simulink model "ProperModel"  (R2024b)
settings: Solver=VariableStepAuto  StartTime=0.0  StopTime=10.0  RelTol=1e-3
values from neighbouring files (symbols this model uses):
  I = diag(Iv)    [InitDoubleSpin.m]    (also in InitLab03.m)
  invI = inv(I)    [InitDoubleSpin.m]    (also in InitLab03.m)
  torque = 0    [InitDoubleSpin.m]
  w0 = [1e-6; 0.005; 0.2]    [InitDoubleSpin.m]    (also in InitLab03.m = [2*pi; 0.5; 1])
  wr0 = 2*pi    (= 6.28318530718)    [InitDoubleSpin.m]
undefined symbols (not defined in the file or in its folder): Js
libraries: matrix_library x1
settings Model: Creator=elisa  LastModifiedBy=filippocamaleonte
settings RTWCC: GPUComputeCapability=3.5

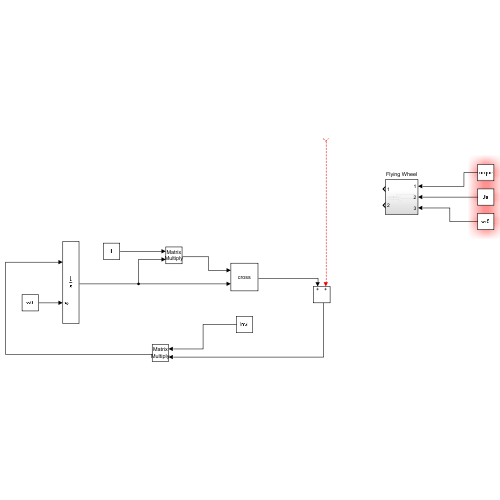
[thumbnail: Simulink's stored preview of the top-level diagram]
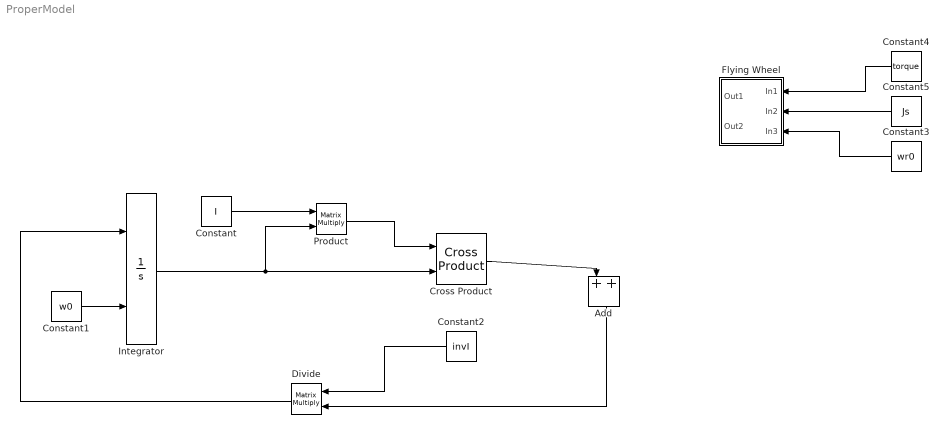
== system ProperModel ==
  Add : Sum
  Constant : Constant  Value=I
  Constant1 : Constant  Value=w0  VectorParams1D=off
  Constant2 : Constant  Value=invI
  Constant3 : Constant  Value=wr0
  Constant4 : Constant  Value=torque
  Constant5 : Constant  Value=Js
  Cross Product : matrix_library/Cross Product
  Divide : Product  Inputs=**  Multiplication=Matrix(*)
  Flying Wheel : Subsystem
  Integrator : Integrator  InitialConditionSource=external
  Product : Product  Multiplication=Matrix(*)
  wires:
  Cross Product/1 -> Add/1
  Add/1 -> Divide/2
  Product/1 -> Cross Product/1
  Constant/1 -> Product/1
  Integrator/1 -> Product/2, Cross Product/2
  Constant1/1 -> Integrator/2
  Constant2/1 -> Divide/1
  Divide/1 -> Integrator/1
  Constant3/1 -> Flying Wheel/3(In3)
  Constant4/1 -> Flying Wheel/1(In1)
  Constant5/1 -> Flying Wheel/2(In2)
  ? -> Add/2

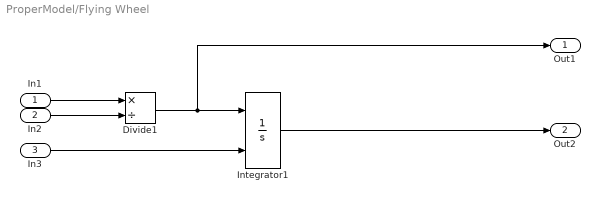
== system ProperModel/Flying Wheel ==
  In1 : Inport
  In2 : Inport  Port=2
  In3 : Inport  Port=3
  Divide1 : Product  Inputs=*/
  Integrator1 : Integrator  InitialConditionSource=external
  Out1 : Outport
  Out2 : Outport  Port=2
  wires:
  Divide1/1 -> Out1/1, Integrator1/1
  In1/1 -> Divide1/1
  Integrator1/1 -> Out2/1
  In3/1 -> Integrator1/2
  In2/1 -> Divide1/2
